simulink model "v2"  (R2023a)
settings: Solver=VariableStepAuto  StartTime=0.0  StopTime=0.5  RelTol=1e-3
settings Model: Creator=user  LastModifiedBy=user

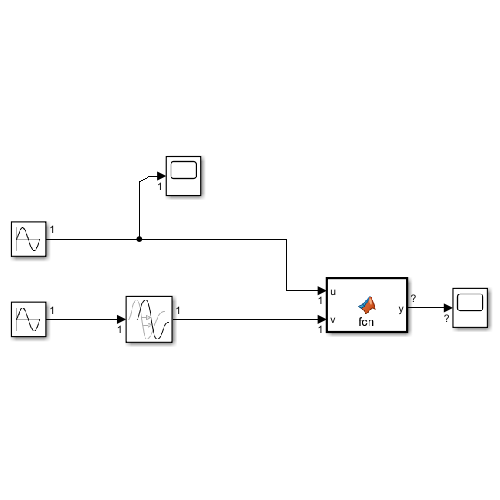
[thumbnail: Simulink's stored preview of the top-level diagram]
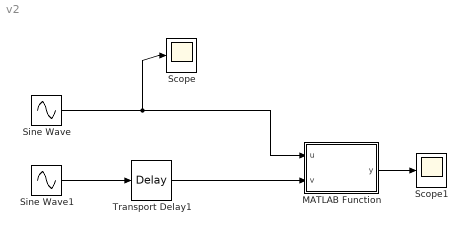
== system v2 ==
  MATLAB Function : MATLAB Function  TreatAsAtomicUnit=on
  Scope : Scope
  Scope1 : Scope
  Sine Wave : Sin  SampleTime=0
  Sine Wave1 : Sin  SampleTime=0
  Transport Delay1 : TransportDelay  DelayTime=0.01
  wires:
  Sine Wave1/1 -> Transport Delay1/1
  Sine Wave/1 -> MATLAB Function/1(u), Scope/1
  Transport Delay1/1 -> MATLAB Function/2(v)
  MATLAB Function/1(y) -> Scope1/1

== matlab function v2/MATLAB Function ==
  data: u input; y output; v input
function y = fcn(u,v)

y=1;
%y=gccphat(u,v)
end
